simulink model "equalizer"  (R2019b)
settings: Solver=VariableStepAuto  StartTime=0.0  StopTime=100  RelTol=1e-3  EnableMultiTasking=on
libraries: dsparch4 x3, dspmathops x3, dspvision x1, dspobslib x1
settings Model: Creator=vladimir_leonidov  LastModifiedBy=andreykorchagin
settings DataIOCC: LimitDataPoints=on  ReturnWorkspaceOutputs=off
settings OptimizationCC: LifeSpan=inf
settings DebuggingCC: AllowSymbolicDim=off  SFUnexpectedBacktrackingDiag=warning  SFNoUnconditionalDefaultTransitionDiag=warning  SFExecutionAtInitializationDiag=none  ArithmeticOperatorsInVariantConditions=warning
settings ModelReferenceCC: PropagateSignalLabelsOutOfModel=off
settings SFSimCC: SimUseLocalCustomCode=off  CustomCodeUndefinedFunction=UseInterfaceOnly
settings RTWCC: RTWUseLocalCustomCode=off
settings CodeAppCC: StateflowObjectComments=on
settings GRTTargetCC: TargetLangStandard=C89/C90 (ANSI)
settings ConfigComp: CovMetricSettings=dw  CovHtmlReporting=on  CovSaveCumulativeToWorkspaceVar=on  CovSaveSingleToWorkspaceVar=on  CovExternalEMLEnable=off

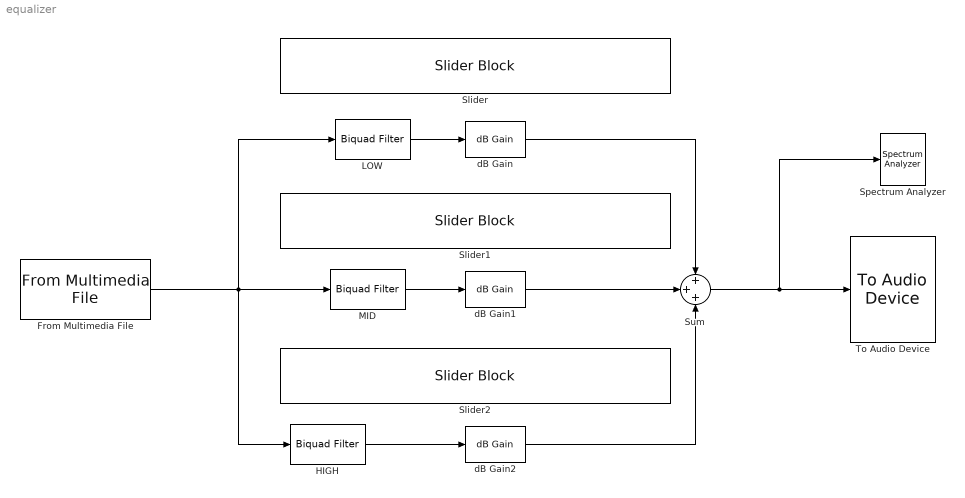
== system equalizer ==
  From Multimedia File : dspvision/From Multimedia File  inputFilename=/Users/andreykorchagin/Desktop/Git/DSP-labs/Lab 3 - Filters/Reports/rock.wav  readRange=[1 Inf]  loop=on  numPlays=inf  outputStreams=Audio only  videoDataType=single  audioDataType=double  inheritSampleTime=on  userDefinedSampleTime=1/30  noAudioOutput=off  isIntensityVideo=off  fourcc=RGB  colorVideoFormat=Separate color signals  outputEOF=off  dataOrg=Column-major  audioFrameSize=1024  computeAudioFrameSize=off  outSamplingMode=Sample based
      settings: SourceProductName=Computer Vision Toolbox  SourceProductBaseCode=VP
  "HIGH " : dsparch4/Biquad Filter  Tag=BlockMethodSubSystem  FilterSource=Dialog parameters  CoeffSource=Specify via dialog  FilterObject=BQF  IIRFiltStruct=Direct form II  BiQuadCoeffs=[1 0 -1 1 0.301281413911877571 0.980368202074170303;1 0 -1 1 1.99839495009804313 0.999372867948402965;1 0 -1 1 0.29553730964998548 0.942245323546703539;1 0 -1 1 1.99714258338279915 0.998119945766865135;1 0 -1 1 0.290067715002303494 0.905581997592033061;1 0 -1 1 1.99589221574618203 0.996869080856208956;1 0 -1 1 0.284858983232886165 0.870308529524853158;1 0 -1 1 1.99464416812852141 0.99562059408726622;1 0 -1 1 0.279898280526321153 0.83635948857498299;1 0 -1 1 1.99339876105019709 0.99437480585168625;1 0 -1 1 0.275173527606570489 0.803673404058536933;1 0 -1 1 1.99215631506536761 0.993132036515899097;1 0 -1 1 0.270673346119282121 0.772192486542578771;1 0 -1 1 1.99091715121142121 0.991892606870726667;1 0 -1 1 0.266387009338989955 0.741862371695368061;1 0 -1 1 1.98968159145348245 0.990656838575966425;1 0 -1 1 0.26230439680751183 0.712631884750180689;1 0 -1 1 1.98844995912349676 0.98942505459946184;1 0 -1 1 0.258415952549814143 0.684452823720438475;1 0 -1 1 1.9872225793531364 0.988197579649925606;1 0 -1 1 0.254712646549054622 0.657279759689937682;1 0 -1 1 1.9859997794999309 0.986974740602910794;1 0 -1 1 1.98478188956590618 0.985756866919218377;1 0 -1 1 0.251185939194223551 0.631069852668260989;1 0 -1 1 1.98356924260790635 0.984544291054924692;1 0 -1 1 0.247827748441936085 0.605782681649111754;1 0 -1 1 1.98236217513887647 0.983337348862307725;1 0 -1 1 0.244630419459162474 0.581380087641594323;1 0 -1 1 0.241586696536259971 0.557826028562407705;1 0 -1 1 1.98116102751917333 0.982136379980752983;1 0 -1 1 1.97996614433688389 0.980941728216612074;1 0 -1 1 0.238689697079768781 0.535086444982609044;1 0 -1 1 1.97877787477633671 0.979753741911221332;1 0 -1 1 0.235932887512567246 0.513129135817193105;1 0 -1 1 1.97759657297337843 0.978572774295645709;1 0 -1 1 0.233310060925287444 0.491923643130620036;1 0 -1 1 1.97642259835655532 0.977399183831315632;1 0 -1 1 0.230815316337339926 0.471441145307674947;1 0 -1 1 1.97525631597266171 0.976233334535001163;1 0 -1 1 0.228443039439198858 0.451654357907404658;1 0 -1 1 1.97409809679543047 0.975075596286942736;1 0 -1 1 0.226187884699310199 0.432537441579715409;1 0 -1 1 1.97294831801576676 0.973926345120511239;1 0 -1 1 0.224044758729738891 0.414065916479517127;1 0 -1 1 1.97180736331204454 0.972785963491974992;1 0 -1 1 0.222008804814273264 0.396216582663523609;1 0 -1 1 1.97067562309874589 0.971654840528609176;1 0 -1 1 0.220075388511393411 0.378967445999906616;1 0 -1 1 1.96955349475162267 0.970533372253399973;1 0 -1 1 0.21824008425251562 0.362297649161889501;1 0 -1 1 1.96844138280752423 0.969421961784460939;1 0 -1 1 0.216498662862862457 0.346187407313234274;1 0 -1 1 1.96733969913690521 0.968321019507195846;1 0 -1 1 0.214847079939004398 0.330617948127071015;1 0 -1 1 1.96624886308692037 0.967230963217158846;1 0 -1 1 0.21328146502282358 0.315571455809736223;1 0 -1 1 1.96516930159285685 0.966152218231326243;1 0 -1 1 0.211798111517065013 0.301031018828855801;1 0 -1 1 1.96410144925579866 0.965085217465758927;1 0 -1 1 0.210393467292487951 0.286980581069787521;1 0 -1 1 1.96304574838396517 0.964030401477049548;1 0 -1 1 0.209064125940968987 0.273404896167261324;1 0 -1 1 1.96200264899553245 0.962988218465423484;1 0 -1 1 0.207806818632982782 0.260289484779675617;1 0 -1 1 1.96097260878027102 0.961959124236840379;1 0 -1 1 0.206618406541459021 0.247620594592323634;1 0 -1 1 1.95995609301769624 0.960943582121792872;1 0 -1 1 0.205495873797349959 0.235385162852920909;1 0 -1 1 1.95895357444909024 0.959942062848203492;1 0 -1 1 0.204436320945218464 0.223570781258503409;1 0 -1 1 1.95796553310094756 0.958955044365978782;1 0 -1 1 0.203436958869867318 0.212165663026993967;1 0 -1 1 1.95699245605735372 0.957983011620755165;1 0 -1 1 0.202495103167496526 0.201158611999874198;1 0 -1 1 1.95603483717892423 0.95702645627447458;1 0 -1 1 0.201608168937058352 0.190538993634320586;1 0 -1 1 1.95509317676593275 0.956085876370466714;1 0 -1 1 0.200773665969500692 0.180296707754184771;1 0 -1 1 1.95416798116345447 0.955161775940833957;1 0 -1 1 ...(+3638 chars)]  ScaleValues=[0.635910453654083052;0.635910453654083052;0.629570420372116302;0.629570420372116302;0.623420250880987625;0.623420250880987625;0.617453244170514282;0.617453244170514282;0.61166303075538353;0.61166303075538353;0.606043553124088197;0.606043553124088197;0.600589047559987543;0.600589047559987543;0.595294027224676059;0.595294027224676059;0.590153266403709242;0.590153266403709242;0.585161785823637648;0.585161785823637648;0.580314838957317725;0.580314838957317725;0.57560789924171063;0.57560789924171063;0.571036648138924852;0.571036648138924852;0.566596963977178292;0.566596963977178292;0.562284911513717955;0.562284911513717955;0.558096732166593945;0.558096732166593945;0.55402883486659571;0.55402883486659571;0.550077787484663072;0.550077787484663072;0.546240308793726648;0.546240308793726648;0.542513260927246721;0.542513260927246721;0.538893642299735687;0.538893642299735687;0.535378580957302286;0.535378580957302286;0.531965328328768416;0.531965328328768416;0.528651253350199468;0.528651253350199468;0.525433836937785559;0.525433836937785559;0.522310666785933519;0.522310666785933519;0.519279432469177182;0.519279432469177182;0.516337920828130903;0.516337920828130903;0.513484011621182179;0.513484011621182179;0.510715673424976258;0.510715673424976258;0.508030959767988843;0.508030959767988843;0.50542800548262945;0.50542800548262945;0.502905023262368522;0.502905023262368522;0.500460300411352033;0.500460300411352033;0.4980921957748633;0.4980921957748633;0.495799136839811139;0.495799136839811139;0.493579616995187376;0.493579616995187376;0.491432192943141444;0.491432192943141444;0.489355482251963014;0.489355482251963014;0.487348161042872763;0.487348161042872763;0.485408961803069972;0.485408961803069972;0.483536671318008759;0.483536671318008759;0.481730128716346462;0.481730128716346462;0.479988223621456267;0.479988223621456267;0.478309894403806612;0.478309894403806612;0.476694126528891537;0.476694126528891537;0.475139950995757288;0.475139950995757288;0.473646442861497208;0.473646442861497208;0.47221271984740032;0.47221271984740032;0.470837941022726525;0.470837941022726525;0.469521305562350277;0.469521305562350277;0.468262051574767635;0.468262051574767635;0.467059454997197698;0.467059454997197698;0.465912828554728597;0.465912828554728597;0.464821520780667907;0.464821520780667907;0.463784915095449057;0.463784915095449057;0.462802428941631094;0.462802428941631094;0.461873512972698907;0.461873512972698907;0.4609976502935344;0.4609976502935344;0.460174355750581743;0.460174355750581743;0.459403175269876118;0.459403175269876118;0.458683685241240091;0.458683685241240091;0.45801549194708352;0.45801549194708352;0.457398231034368052;0.457398231034368052;0.456831567028410213;0.456831567028410213;0.456315192887317089;0.456315192887317089;0.455848829595948191;0.455848829595948191;0.455432225798407753;0.455432225798407753;0.455065157468165449;0.455065157468165449;0.454747427615002975;0.454747427615002975;0.454478866028075024;0.454478866028075024;0.454259329054463423;0.454259329054463423;0.454088699412690977;0.454088699412690977;0.453966886040746975;0.453966886040746975;0.453893823978259836;0.453893823978259836;0.453869474282535379;1]  IC=0  ICnum=0  ICden=0  a0Flag=Warning  optimizeScaleValues=on  ScaleValueMode=Specify via input port (g)  InputProcessing=Columns as channels (frame based)  roundingMode=Floor  overflowMode=off  scaleValueFracLength=14  denProdOutputFracLength=30  denAccumFracLength=30  secondMemoryFracLength=15
      settings: SourceProductName=DSP System Toolbox
  LOW : dsparch4/Biquad Filter  Tag=BlockMethodSubSystem  FilterSource=Dialog parameters  CoeffSource=Specify via dialog  FilterObject=BQF  IIRFiltStruct=Direct form II  BiQuadCoeffs=[1 0 -1 1 -1.97606379204297267 0.990077885036462435;1 0 -1 1 -1.99647100310135572 0.997415351169754771;1 0 -1 1 -1.95715363139769183 0.97081557346782732;1 0 -1 1 -1.99126511756397728 0.992221985969370612;1 0 -1 1 -1.93966165960929571 0.952773561057095986;1 0 -1 1 -1.98593521472952195 0.986920567363905432;1 0 -1 1 -1.92406918592910525 0.936449397953399543;1 0 -1 1 -1.98037912378226677 0.981411272374218435;1 0 -1 1 -1.91082348166437033 0.922308379667510114;1 0 -1 1 -1.97447458473882742 0.975576028790520633;1 0 -1 1 -1.90035320796481599 0.910798557172385226;1 0 -1 1 -1.96806586899532876 0.969266110051015373;1 0 -1 1 -1.96094423277616081 0.962284477310347497;1 0 -1 1 -1.89309117639226132 0.902373521328127759;1 0 -1 1 -1.95282088597207815 0.954362467768732126;1 0 -1 1 -1.88950514798673908 0.897524311458319013;1 0 -1 1 -1.94330373722105865 0.945143852743445256;1 0 -1 1 -1.89012490596877702 0.896810688475649709;1 0 -1 1 -1.93196146320243001 0.934261292255661679;1 0 -1 1 -1.89548165990111905 0.900813590191788416;1 0 -1 1 -1.91882097621496017 0.921838538862183587;1 0 -1 1 -1.90561341468234691 0.909670456961579443]  ScaleValues=[0.0439184123509175073;0.0439184123509175073;0.0436496146001236623;0.0436496146001236623;0.0433937083217029035;0.0433937083217029035;0.0431552105435565742;0.0431552105435565742;0.0429381054821255381;0.0429381054821255381;0.042745835229254181;0.042745835229254181;0.0425813043020621673;0.0425813043020621673;0.0424468929842843345;0.0424468929842843345;0.0423444750267275849;0.0423444750267275849;0.0422754360388461828;0.0422754360388461828;0.0422406897006661411;0.0422406897006661411;1]  IC=0  ICnum=0  ICden=0  a0Flag=Warning  optimizeScaleValues=on  ScaleValueMode=Specify via input port (g)  InputProcessing=Columns as channels (frame based)  roundingMode=Floor  overflowMode=off  scaleValueFracLength=14  denProdOutputFracLength=30  denAccumFracLength=30  secondMemoryFracLength=15
      settings: SourceProductName=DSP System Toolbox
  MID : dsparch4/Biquad Filter  Tag=BlockMethodSubSystem  FilterSource=Dialog parameters  CoeffSource=Specify via dialog  FilterObject=BQF  IIRFiltStruct=Direct form II  BiQuadCoeffs=[1 0 -1 1 0.195273526082052118 0.980398752336620882;1 0 -1 1 -1.97254236364563051 0.99690688074820677;1 0 -1 1 0.191302736522291073 0.942330435171554348;1 0 -1 1 -1.96645410714352109 0.990748941494883906;1 0 -1 1 0.187269777948425364 0.905708779042088019;1 0 -1 1 -1.96039692324285997 0.984627928464470892;1 0 -1 1 0.183178787304100865 0.870459777764320597;1 0 -1 1 -1.95436992233725526 0.978542895375558164;1 0 -1 1 0.179033581294258837 0.836514395687351642;1 0 -1 1 -1.94837223794075198 0.97249292214410421;1 0 -1 1 0.174837686317568852 0.803808177146861702;1 0 -1 1 -1.94240302911850415 0.96647711724055585;1 0 -1 1 0.170594365872560383 0.772280891999391983;1 0 -1 1 -1.93646148293514297 0.96049462005145736;1 0 -1 1 0.166306645729297153 0.741876213500599402;1 0 -1 1 -1.93054681694769315 0.95454460327237034;1 0 -1 1 -1.92465828176984077 0.94862627535855637;1 0 -1 1 0.161977337127730686 0.712541425224014646;1 0 -1 1 -1.9187951637345233 0.942738883059879296;1 0 -1 1 0.15760905823723817 0.684227154095103707;1 0 -1 1 -1.91295678768221511 0.936881714066570948;1 0 -1 1 0.153204254088928404 0.65688712694641016;1 0 -1 1 -1.90714251990302697 0.93105409979302145;1 0 -1 1 0.148765215172438681 0.630477948289632661;1 0 -1 1 -1.90135177126164678 0.925255418327429413;1 0 -1 1 0.144294094871833173 0.604958897255224559;1 0 -1 1 -1.89558400053526599 0.919485097576066335;1 0 -1 1 0.139792925900608545 0.58029174187405852;1 0 -1 1 -1.88983871799621372 0.913742618632185533;1 0 -1 1 0.135263635883276973 0.556440569073176183;1 0 -1 1 -1.8841154892724945 0.90802751940088422;1 0 -1 1 0.130708062220350807 0.53337162893178014;1 0 -1 1 -1.87841393952156555 0.902339398513029689;1 0 -1 1 0.126127966364616761 0.511053191897645087;1 0 -1 1 -1.87273375795461927 0.896677919563060977;1 0 -1 1 0.121525047629129607 0.489455417800557291;1 0 -1 1 0.116900956641251136 0.468550235620188382;1 0 -1 1 -1.86707470275129461 0.891042815707762781;1 0 -1 1 -1.86143660640713726 0.885433894665228705;1 0 -1 1 0.112257308552134172 0.448311233073326876;1 0 -1 1 -1.85581938155915371 0.87985104415587323;1 0 -1 1 0.107595696107123051 0.42871355518087817;1 0 -1 1 -1.85022302733772159 0.87429423782989657;1 0 -1 1 0.102917702679689221 0.409733811060067121;1 0 -1 1 -1.84464763629640549 0.868763541728524102;1 0 -1 1 0.0982249153693045274 0.391349988263196336;1 0 -1 1 -1.83909340197446514 0.863259121329138734;1 0 -1 1 0.0935189382622479415 0.373541374051926833;1 0 -1 1 -1.83356062715020718 0.857781249227379639;1 0 -1 1 0.0888014059534268652 0.356288483056543981;1 0 -1 1 -1.82804973284666561 0.85233031351216082;1 0 -1 1 0.084073997426784064 0.339572990823642729;1 0 -1 1 -1.82256126815415476 0.846906826892200981;1 0 -1 1 0.0793384503916012424 0.32337767280384383;1 0 -1 1 -1.81709592093711736 0.841511436635054899;1 0 -1 1 0.0745965761717298365 0.307686348374199004;1 0 -1 1 -1.81165452949491113 0.836144935381492149;1 0 -1 1 0.0698502752443810326 0.292483829528152883;1 0 -1 1 -1.80623809524771639 0.830808272899166922;1 0 -1 1 0.0651015535240385412 0.277755873899864336;1 0 -1 1 -1.80084779651902971 0.825502568839553086;1 0 -1 1 0.0603525394852791608 0.263489141819537975;1 0 -1 1 -1.79548500348513151 0.820229126560744315;1 0 -1 1 0.055605502215070185 0.249671157122463294;1 0 -1 1 -1.79015129435856446 0.814989448075356226;1 0 -1 1 0.0508628704800384995 0.236290271456838175;1 0 -1 1 -1.78484847286673087 0.809785250176878302;1 0 -1 1 0.0461272528866595033 0.223335631854217287;1 0 -1 1 -1.77957858707725114 0.804618481788732298;1 0 -1 1 0.0414014592012783428 0.210797151341590217;1 0 -1 1 -1.77434394960762898 0.799491342566911567;1 0 -1 1 0.0366885228816115211 0.198665482385590203;1 0 -1 1 -1.76914715923729693 0.794406302768662864;1 0 -1 1 0.0319917248504999752 0.186931992966919758;1 0 -1 1 -1.76399112391323998 0.789366124374539013;1 0 -1 1 0.0273146185149075252 0.175588745086567549;1 0 -1 1 -1.75887908510519475 0.784373883418238993;1 0 -1 1 0.0226610559968068656 0.164628475504504074;1 0 -1 1 ...(+3079 chars)]  ScaleValues=[0.6825594232324107;0.6825594232324107;0.674965650926226401;0.674965650926226401;0.667625519098444919;0.667625519098444919;0.66052895947695256;0.66052895947695256;0.653666465270462793;0.653666465270462793;0.647029053625218342;0.647029053625218342;0.640608231081056134;0.640608231081056134;0.634395961752130644;0.634395961752130644;0.628384637985993089;0.628384637985993089;0.622567053279874383;0.622567053279874383;0.616936377255320134;0.616936377255320134;0.611486132512128022;0.611486132512128022;0.606210173200153246;0.606210173200153246;0.601102665163245065;0.601102665163245065;0.596158067523570145;0.596158067523570145;0.591371115587090879;0.591371115587090879;0.586736804962157521;0.586736804962157521;0.582250376793194357;0.582250376793194357;0.577907304020455981;0.577907304020455981;0.573703278584908771;0.573703278584908771;0.569634199504555405;0.569634199504555405;0.565696161755066651;0.565696161755066651;0.561885445893480107;0.561885445893480107;0.558198508369055157;0.558198508369055157;0.554631972470182366;0.554631972470182366;0.551182619860602907;0.551182619860602907;0.547847382662136506;0.547847382662136506;0.544623336044696704;0.544623336044696704;0.541507691287616555;0.541507691287616555;0.538497789279259953;0.538497789279259953;0.535591094424583192;0.535591094424583192;0.532785188932752618;0.532785188932752618;0.530077767459154248;0.530077767459154248;0.527466632078172126;0.527466632078172126;0.524949687564963186;0.524949687564963186;0.522524936966163978;0.522524936966163978;0.520190477441017873;0.520190477441017873;0.517944496355837947;0.517944496355837947;0.515785267616032272;0.515785267616032272;0.513711148221117297;0.513711148221117297;0.511720575029250502;0.511720575029250502;0.509812061718833087;0.509812061718833087;0.507984195935665683;0.507984195935665683;0.506235636615008811;0.506235636615008811;0.504565111468692651;0.504565111468692651;0.502971414628164082;0.502971414628164082;0.501453404435034278;0.501453404435034278;0.500010001371330448;0.500010001371330448;0.498640186122235596;0.498640186122235596;0.497342997764649852;0.497342997764649852;0.496117532075412593;0.496117532075412593;0.494962939953498715;0.494962939953498715;0.493878425950942501;0.493878425950942501;0.492863246907658037;0.492863246907658037;0.491916710685709135;0.491916710685709135;0.491038174998948085;0.491038174998948085;0.490227046334281824;0.490227046334281824;0.489482778961147891;0.489482778961147891;0.488804874026087743;0.488804874026087743;0.488192878729591551;0.488192878729591551;0.487646385582665653;0.487646385582665653;0.487165031740834864;0.487165031740834864;0.486748498413540509;0.486748498413540509;0.486396510347138211;0.486396510347138211;0.486108835379928328;0.486108835379928328;0.485885284067877343;0.485885284067877343;0.485725709379905168;0.485725709379905168;0.485630006461824915;0.485630006461824915;0.485598112468229814;1]  IC=0  ICnum=0  ICden=0  a0Flag=Warning  optimizeScaleValues=on  ScaleValueMode=Specify via input port (g)  InputProcessing=Columns as channels (frame based)  roundingMode=Floor  overflowMode=off  scaleValueFracLength=14  denProdOutputFracLength=30  denAccumFracLength=30  secondMemoryFracLength=15
      settings: SourceProductName=DSP System Toolbox
  Slider : SliderBlock  ScaleMin=-100
  Slider1 : SliderBlock  ScaleMin=-100
  Slider2 : SliderBlock  ScaleMin=-100
  Spectrum Analyzer : SpectrumAnalyzer
  Sum : Sum  Inputs=+++
  To Audio Device : dspobslib/To Audio Device  deviceName=Default  inheritSampleRate=on  sampleRate=44100  deviceDatatype=Determine from input data type  autoBufferSize=on  bufferSize=4096  queueDuration=1.0  defaultOutputChannelMapping=on  outputChannelMapping=1:2  outputNumUnderrunSamples=off
      settings: SourceProductName=DSP System Toolbox  SourceProductBaseCode=DS
  dB Gain : dspmathops/dB Gain  dB=0  intype=Amplitude
      settings: SourceProductName=DSP System Toolbox  SourceProductBaseCode=DS
  dB Gain1 : dspmathops/dB Gain  dB=0  intype=Amplitude
      settings: SourceProductName=DSP System Toolbox  SourceProductBaseCode=DS
  dB Gain2 : dspmathops/dB Gain  dB=0  intype=Amplitude
      settings: SourceProductName=DSP System Toolbox  SourceProductBaseCode=DS
  wires:
  dB Gain/1 -> Sum/1
  dB Gain1/1 -> Sum/2
  dB Gain2/1 -> Sum/3
  Sum/1 -> Spectrum Analyzer/1, To Audio Device/1
  "HIGH "/1 -> dB Gain2/1
  MID/1 -> dB Gain1/1
  LOW/1 -> dB Gain/1
  From Multimedia File/1 -> "HIGH "/1, LOW/1, MID/1
